simulink library "cvt_powertrain_lib"  (R2026a)
settings: Solver=VariableStepAuto
undefined symbols (not defined in the file or in its folder): fluids, HMPST
libraries: fl_lib x90, nesl_utility x31, cvt_components_lib x27, sdl_lib x24, SimscapeFluids_lib x11, simulink_extras x6, $bdroot x4, ee_lib x2, batteryecm_lib x1, simulink x1, engine_mgmt_lib x1, slpidlib x1
(part 4 of 4)

== system cvt_powertrain_lib/Controller/Desired Ratio Calc/MB Control ==
  note: No filter here - brake needs to release right away.
  Decel Error : Inport
  wTransOutCmd : Inport  Port=2
  Rset : Inport  Port=3
  AccumLimUp : Inport  Port=4
  HRBPowerLim : Inport  Port=5
  Add1 : Sum  Inputs=+++
  Compare To Constant : simulink/Logic and Bit Operations/Compare To Constant  relop=<=  const=0.02  OutDataTypeStr=boolean
  Data Type Conversion : DataTypeConversion  OutDataTypeStr=double  SaturateOnIntegerOverflow=off  RndMeth=Floor
  PI MB No HRB : Subsystem
  PI MB with MRB : Subsystem
  Product3 : Product  Inputs=3
  Product4 : Product
  Transfer Fcn (with initial outputs)1 : simulink_extras/Additional Linear/Transfer Fcn (with initial outputs)  N=1  D=[HMPST.MB.Control.tFilt 1]  Y0=1  U0=1
  Transfer Fcn (with initial outputs)2 : simulink_extras/Additional Linear/Transfer Fcn (with initial outputs)  N=1  D=[HMPST.MB.Control.tFilt 1]  Y0=1  U0=1
  MBCtrl (-) : Outport
  wires:
  Transfer Fcn (with initial outputs)1/1 -> Add1/3
  Transfer Fcn (with initial outputs)2/1 -> Add1/2
  HRBPowerLim/1 -> Product4/2
  AccumLimUp/1 -> Product3/3
  wTransOutCmd/1 -> Compare To Constant/1
  PI MB with MRB/1(ctrl) -> Transfer Fcn (with initial outputs)1/1
  Add1/1 -> MBCtrl (-)/1
  Product4/1 -> PI MB with MRB/1(error)
  PI MB No HRB/1(ctrl) -> Transfer Fcn (with initial outputs)2/1
  Data Type Conversion/1 -> Add1/1
  Compare To Constant/1 -> Data Type Conversion/1
  Rset/1 -> PI MB with MRB/2(Rset), PI MB No HRB/2(Rset), Product3/2
  Product3/1 -> PI MB No HRB/1(error)
  Decel Error/1 -> Product4/1, Product3/1

== system cvt_powertrain_lib/Controller/Desired Ratio Calc/VehSpdDir ==
  u : Inport
  Constant1 : Constant
  Constant2 : Constant  Value=-1
  Constant3 : Constant  Value=0
  Gain : Gain  Gain=-1
  Switch : Switch  Criteria=u2 > Threshold  Threshold=0.001  SaturateOnIntegerOverflow=off  InputSameDT=off
  Switch1 : Switch  Criteria=u2 > Threshold  Threshold=0.001  SaturateOnIntegerOverflow=off  InputSameDT=off
  u_dir : Outport
  wires:
  Gain/1 -> Switch1/2
  Switch/1 -> u_dir/1
  u/1 -> Switch/2, Gain/1
  Constant1/1 -> Switch/1
  Switch1/1 -> Switch/3
  Constant3/1 -> Switch1/3
  Constant2/1 -> Switch1/1

== system cvt_powertrain_lib/Controller/Desired Ratio Calc/HRB Control/PI HRB Brake ==
  error : Inport
  Rset : Inport  Port=2
  Gain : Gain  Gain=0.02*0.2
  Gain3 : Gain  Gain=0.002+0.0005
  Integrator : Integrator  ExternalReset=falling
  Sum : Sum  Inputs=++|
  ctrl : Outport
  wires:
  Rset/1 -> Integrator/2
  Integrator/1 -> Sum/1
  error/1 -> Gain3/1, Gain/1
  Sum/1 -> ctrl/1
  Gain3/1 -> Integrator/1
  Gain/1 -> Sum/2

== system cvt_powertrain_lib/Controller/Desired Ratio Calc/HRB Control/PI HRB Regen ==
  error : Inport
  Rset : Inport  Port=2
  Gain : Gain  Gain=0.01*0.2
  Gain3 : Gain  Gain=0.001
  Integrator : Integrator  ExternalReset=falling
  Sum : Sum  Inputs=++|
  ctrl : Outport
  wires:
  Gain/1 -> Sum/2
  Gain3/1 -> Integrator/1
  Sum/1 -> ctrl/1
  error/1 -> Gain/1, Gain3/1
  Integrator/1 -> Sum/1
  Rset/1 -> Integrator/2

== system cvt_powertrain_lib/Controller/Desired Ratio Calc/MB Control/PI MB No HRB ==
  error : Inport
  Rset : Inport  Port=2
  Gain : Gain  Gain=HMPST.MB.Control.NoHRB.Kp
  Gain3 : Gain  Gain=HMPST.MB.Control.NoHRB.Ki
  Integrator : Integrator  ExternalReset=falling
  Sum : Sum  Inputs=++|
  ctrl : Outport
  wires:
  Rset/1 -> Integrator/2
  Integrator/1 -> Sum/1
  error/1 -> Gain3/1, Gain/1
  Sum/1 -> ctrl/1
  Gain3/1 -> Integrator/1
  Gain/1 -> Sum/2

== system cvt_powertrain_lib/Controller/Desired Ratio Calc/MB Control/PI MB with MRB ==
  error : Inport
  Rset : Inport  Port=2
  Gain : Gain  Gain=HMPST.MB.Control.WithHRB.Kp
  Gain3 : Gain  Gain=HMPST.MB.Control.WithHRB.Ki
  Integrator : Integrator  ExternalReset=falling
  Sum : Sum  Inputs=++|
  ctrl : Outport
  wires:
  Gain/1 -> Sum/2
  Gain3/1 -> Integrator/1
  Sum/1 -> ctrl/1
  error/1 -> Gain/1, Gain3/1
  Integrator/1 -> Sum/1
  Rset/1 -> Integrator/2

== stateflow chart cvt_powertrain_lib/Controller/CVT Ratio Ctrl/Clutch Truth Table ==
  state ClutchLogic
    during:
    [K1Actv,K2Actv,K3Actv,K4Actv,KbActv] = ClutchTable(Range);
    state Rest
      during:
      KvActv = 0;
      KrActv = 0;
    state Fwd
      during:
      KvActv = 1;
      KrActv = 0;
    state Rev
      during:
      KvActv = 0;
      KrActv = 1;
    (default) -> (junction 53)
    (junction 53) -> Fwd [order 3]
    (junction 53) -> Rev [order 2] : [CmdVehSpdDir==-1]
    (junction 53) -> Rest [order 1] : [CmdVehSpdDir==0]
    Fwd -> Rest : [CmdVehSpdDir~=1]
    Rev -> Rest : [CmdVehSpdDir~=-1]
    Rest -> Fwd [order 1] : [CmdVehSpdDir==1]
    Rest -> Rev [order 2] : [CmdVehSpdDir==-1]
  data: R function_input; K1 function_output; K2 function_output; K3 function_output; K4 function_output; Kb function_output; Range input; K1Actv output; K2Actv output; K3Actv output; K4Actv output; KbActv output; KvActv output; KrActv output; CmdVehSpdDir input
  function [K1,K2,K3,K4,Kb] = ClutchTable(R):
    | function [K1,K2,K3,K4,Kb] = ClutchTable(R)
    | 
    | aVarTruthTableCondition_1 = false;
    | aVarTruthTableCondition_2 = false;
    | aVarTruthTableCondition_3 = false;
    | aVarTruthTableCondition_4 = false;
    | 
    | 
    | % Range1
    | 
    | aVarTruthTableCondition_1 = logical(R == 1);
    | 
    | % Range2
    | 
    | aVarTruthTableCondition_2 = logical(R == 2);
    | 
    | % Range3
    | 
    | aVarTruthTableCondition_3 = logical(R == 3);
    | 
    | % Range4
    | 
    | aVarTruthTableCondition_4 = logical(R == 4);
    | 
    | if (aVarTruthTableCondition_1 && ~aVarTruthTableCondition_2 && ~aVarTruthTableCondition_3 && ~aVarTruthTableCondition_4)
    |     A1();
    | elseif (~aVarTruthTableCondition_1 && aVarTruthTableCondition_2 && ~aVarTruthTableCondition_3 && ~aVarTruthTableCondition_4)
    |     A2();
    | elseif (~aVarTruthTableCondition_1 && ~aVarTruthTableCondition_2 && aVarTruthTableCondition_3 && ~aVarTruthTableCondition_4)
    |     A3();
    | elseif (~aVarTruthTableCondition_1 && ~aVarTruthTableCondition_2 && ~aVarTruthTableCondition_3 && aVarTruthTableCondition_4)
    |     A4();
    | else % Default
    |     A5();
    | end
    | 
    | function A1()
    | 
    | % ClutchCtrlR1
    | 
    | K1 = 1; K2 = 0; K3 = 0; K4 = 0; Kb = 1;
    | 
    | function A2()
    | 
    | % ClutchCtrlR2
    | 
    | K1 = 0; K2 = 1; K3 = 0; K4 = 0; Kb = 1;
    | 
    | function A3()
    | 
    | % ClutchCtrlR3
    | 
    | K1 = 0; K2 = 1; K3 = 1; K4 = 0; Kb = 0;
    | 
    | function A4()
    | 
    | % ClutchCtrlR4
    | 
    | K1 = 0; K2 = 1; K3 = 0; K4 = 1; Kb = 0;
    | 
    | function A5()
    | 
    | % Default
    | 
    | K1 = 0; K2 = 0; K3 = 0; K4 = 0; Kb = 0;
